simulink model "part1"  (R2024a)
settings: Solver=VariableStepAuto  StartTime=0.0  StopTime=200  RelTol=1e-3
undefined symbols (not defined in the file or in its folder): magnitude
settings Model: Creator=katutu  LastModifiedBy=katutu

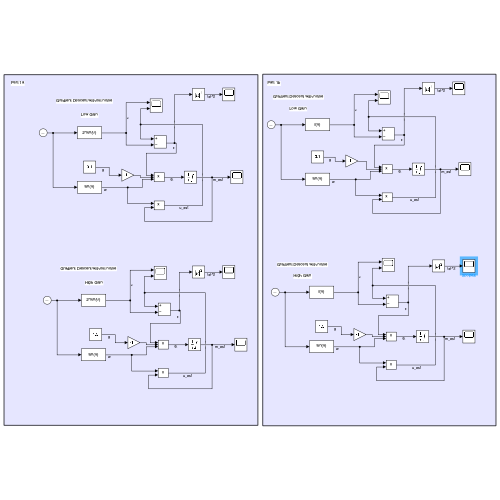
[thumbnail: Simulink's stored preview of the top-level diagram]
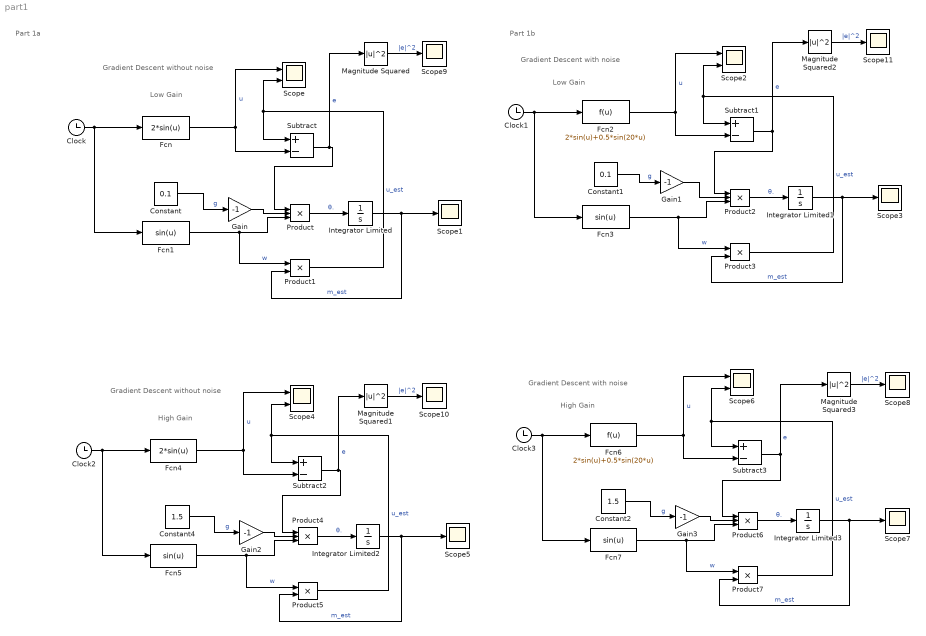
== system part1 ==
  note: Part 1a
  note: Low Gain
  note: Gradient Descent without noise
  note: Gradient Descent with noise
  note: Low Gain
  note: High Gain
  note: Gradient Descent with noise
  note: High Gain
  note: Gradient Descent without noise
  note: Part 1b
  Clock{,1..3} (4 alike) : Clock
  Constant : Constant  Value=0.1
  Constant1 : Constant  Value=0.1
  Constant2 : Constant  Value=1.5
  Constant4 : Constant  Value=1.5
  Fcn : Fcn  Expr=2*sin(u)
  Fcn{1,3,5,7} (4 alike) : Fcn  Expr=sin(u)
  Fcn2 : Fcn  Expr=2*sin(u)+0.5*sin(20*u)
  Fcn4 : Fcn  Expr=2*sin(u)
  Fcn6 : Fcn  Expr=2*sin(u)+0.5*sin(20*u)
  Gain{,1..3} (4 alike) : Gain  Gain=-1
  Integrator Limited{,1..3} (4 alike) : Integrator  LimitOutput=on  UpperSaturationLimit=10  LowerSaturationLimit=0
  Magnitude Squared{,1..3} (4 alike) : Math  Operator=magnitude^2
  Product{,2,4,6} (4 alike) : Product  Inputs=3
  Product{1,3,5,7} (4 alike) : Product
  Scope{,2,4,6} (4 alike) : Scope  NumInputPorts=2
  Scope{1,3,5,7..11} (8 alike) : Scope
  Subtract{,1..3} (4 alike) : Sum  Inputs=+-
  wires:
  Fcn/1 -> Subtract/2, Scope/1  "u"
  Clock/1 -> Fcn1/1, Fcn/1
  Fcn1/1 -> Product1/1, Product/3  "w"
  Subtract/1 -> Magnitude Squared/1, Product/1  "e"
  Product/1 -> Integrator Limited/1  "θ."
  Integrator Limited/1 -> Product1/2, Scope1/1  "m_est"
  Product1/1 -> Subtract/1, Scope/2  "u_est"
  Integrator Limited1/1 -> Scope3/1, Product3/2  "m_est"
  Product2/1 -> Integrator Limited1/1  "θ."
  Product3/1 -> Subtract1/1, Scope2/2  "u_est"
  Fcn2/1 -> Subtract1/2, Scope2/1  "u"
  Clock1/1 -> Fcn3/1, Fcn2/1
  Fcn3/1 -> Product3/1, Product2/3  "w"
  Fcn6/1 -> Subtract3/2, Scope6/1  "u"
  Product6/1 -> Integrator Limited3/1  "θ."
  Integrator Limited2/1 -> Product5/2, Scope5/1  "m_est"
  Product4/1 -> Integrator Limited2/1  "θ."
  Product7/1 -> Subtract3/1, Scope6/2  "u_est"
  Subtract3/1 -> Magnitude Squared3/1, Product6/1  "e"
  Clock2/1 -> Fcn5/1, Fcn4/1
  Product5/1 -> Subtract2/1, Scope4/2  "u_est"
  Clock3/1 -> Fcn7/1, Fcn6/1
  Fcn7/1 -> Product7/1, Product6/3  "w"
  Integrator Limited3/1 -> Product7/2, Scope7/1  "m_est"
  Fcn4/1 -> Subtract2/2, Scope4/1  "u"
  Subtract2/1 -> Magnitude Squared1/1, Product4/1  "e"
  Fcn5/1 -> Product5/1, Product4/3  "w"
  Gain/1 -> Product/2
  Constant/1 -> Gain/1  "g"
  Gain1/1 -> Product2/2
  Constant1/1 -> Gain1/1  "g"
  Gain2/1 -> Product4/2
  Constant4/1 -> Gain2/1  "g"
  Gain3/1 -> Product6/2
  Constant2/1 -> Gain3/1  "g"
  Magnitude Squared/1 -> Scope9/1  "|e|^2"
  Magnitude Squared1/1 -> Scope10/1  "|e|^2"
  Magnitude Squared2/1 -> Scope11/1  "|e|^2"
  Subtract1/1 -> Magnitude Squared2/1, Product2/1  "e"
  Magnitude Squared3/1 -> Scope8/1  "|e|^2"
